simulink model "Cau_1_PCM_vs_KhoiPhucPCM"  (R2019a)
settings: Solver=VariableStepAuto  StartTime=0.0  StopTime=10.0  RelTol=1e-3
libraries: dspquant2 x2, commutil2 x2, dsparch4 x1, dspsigops x1
settings Model: Creator=Thanh_Hai  LastModifiedBy=Thanh_Hai

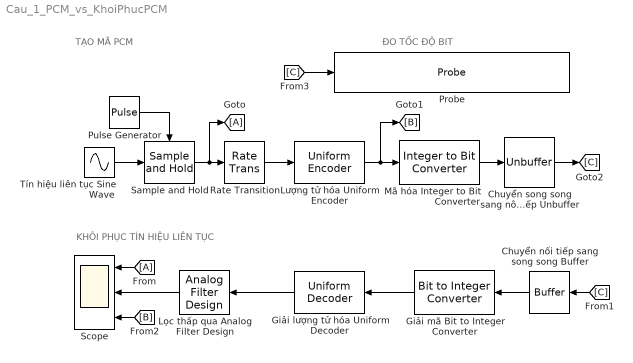
== system Cau_1_PCM_vs_KhoiPhucPCM ==
  note: TẠO MÃ PCM
  note: KHÔI PHỤC TÍN HIỆU LIÊN TỤC
  note: ĐO TỐC ĐỘ BIT
  Chuyển nối tiếp sang song song Buffer : Buffer  N=3  OutputFrames=off
  Chuyển song song sang nôi tiếp Unbuffer : Unbuffer
  Giải lượng tử hóa Uniform Decoder : dspquant2/Uniform Decoder  peak=1  bits=3  overflowMode=Saturate  otype=Double
      settings: SourceProductName=DSP System Toolbox  SourceProductBaseCode=DS
  Giải mã Bit to Integer Converter : commutil2/Bit to Integer Converter  nbits=3  bitOrder=MSB first  signedOutputValues=Unsigned  outDtype=Inherit via internal rule  outDtypeSigned=Inherit via internal rule
      settings: SourceProductName=Communications Toolbox
  Lượng tử hóa Uniform Encoder : dspquant2/Uniform Encoder  peak=1  bits=3  otype=Unsigned integer
      settings: SourceProductName=DSP System Toolbox
  Lọc thấp qua Analog Filter Design : dsparch4/Analog Filter Design  method=Butterworth  filttype=Lowpass  N=12  Wlo=2*pi*4000  Whi=80  Rp=2  Rs=40
  Mã hóa Integer to Bit Converter : commutil2/Integer to Bit Converter  nbits=3  signedInputValues=Unsigned  bitOrder=MSB first  outDtype=Inherit via internal rule
      settings: SourceProductName=Communications Toolbox
  Probe : Probe  ProbeSignalDimensions=on
  Pulse Generator : DiscretePulseGenerator  PulseType=Time based  Period=1/8000  PulseWidth=50
  Rate Transition : RateTransition  OutPortSampleTime=1/8000
  Sample and Hold : dspsigops/Sample and Hold  trig=Rising edge  initCond=0  latchinput=off
  Scope : Scope  NumInputPorts=3
  Tín hiệu liên tục Sine Wave : Sin  Frequency=2*pi*3000  SampleTime=1/100000
  wires:
  Tín hiệu liên tục Sine Wave/1 -> Sample and Hold/1
  Lượng tử hóa Uniform Encoder/1 -> [B], Mã hóa Integer to Bit Converter/1
  Mã hóa Integer to Bit Converter/1 -> Chuyển song song sang nôi tiếp Unbuffer/1
  Pulse Generator/1 -> Sample and Hold/Trigger
  Sample and Hold/1 -> [A], Rate Transition/1
  Rate Transition/1 -> Lượng tử hóa Uniform Encoder/1
  Chuyển song song sang nôi tiếp Unbuffer/1 -> [C]
  Chuyển nối tiếp sang song song Buffer/1 -> Giải mã Bit to Integer Converter/1
  Giải mã Bit to Integer Converter/1 -> Giải lượng tử hóa Uniform Decoder/1
  Giải lượng tử hóa Uniform Decoder/1 -> Lọc thấp qua Analog Filter Design/1
  [A] -> Scope/1
  Lọc thấp qua Analog Filter Design/1 -> Scope/2
  [C] -> Chuyển nối tiếp sang song song Buffer/1
  [B] -> Scope/3
  [C] -> Probe/1
